simulink model "Aearial_Inspection_UAV_Simulation"  (R2023a)
settings: Solver=daessc  StartTime=0.0  StopTime=tf  MaxStep=0.1  MinStep=1e-30  RelTol=1e-4
values from neighbouring files (symbols this model uses):
  arm_start = 0    [InitScript.m]
  X = T*[x0;y0]    [line2circle.m]
undefined symbols (not defined in the file or in its folder): arm_end, DiscIntNeverNeededParam, F, is_gust_active, Light, MIL, Mode, Motor_data, params, Robotic_Arm_ASM_DataFile, Sensor_err, servo_specs, simple_env, stepper, Tm, wind_speed, xStack1, xStack2, Y, Z
libraries: sm_lib x399, nesl_utility x78, simulink x25, dspsrcs4 x16, simulink_extras x8, sharedtransform x7, aerolibwind2 x2, sharedutil x1
(part 12 of 12)

== matlab function Aearial_Inspection_UAV_Simulation/Path Palnner/Arm Guid/Senario 2/senario_2 ==
  data: t input; desired_pos output; desired_psi output
function [desired_pos,desired_psi] = senario_2(t)

desired_psi = [0 0 0];
desired_pos = [0 0 0];


end

== matlab function Aearial_Inspection_UAV_Simulation/Path Palnner/Arm Guid/Senario 3/senario_3 ==
  data: t input; desired_pos output; desired_psi output
function [desired_pos,desired_psi] = senario_3(t)

desired_psi = [0 0 0];
desired_pos = [0 0 0];


end

== matlab function Aearial_Inspection_UAV_Simulation/Path Palnner/Arm Guid/Senario 4/senario_1 ==
  data: t input; desired_pos output; desired_psi output
function [desired_pos,desired_psi] = senario_4(t)

desired_psi = 0;
desired_pos = [0 0 0];


end

== matlab function Aearial_Inspection_UAV_Simulation/Path Palnner/Arm Guid/Senario 5/senario_5 ==
  data: t input; desired_pos output; desired_psi output; ArmMode input; arm_start parameter; uav_pos input; params parameter
function [desired_pos, desired_psi] = senario_5(t, ArmMode, arm_start, uav_pos, params)
x = uav_pos(1)+0.03;
y = uav_pos(2);
z = uav_pos(3);

start_z = 0.35;
start_x = 1;


lift_up_time = params.t_arm_lift_up;
wait_time    = params.t_arm_wait;
forward_time = params.t_arm_forward_time;
keep_time = params.t_inspection;
backward_time = params.t_probe_backward;
down_time = params.t_probe_down;

if ArmMode == 1
    t = t - arm_start;
    desired_psi = 0;
    if(t<lift_up_time)
        desired_pos = [start_x -y t*(-z-start_z)/lift_up_time+start_z];
    elseif (t < lift_up_time + wait_time)
        desired_pos = [start_x -y -z];
    elseif (t<forward_time+lift_up_time + wait_time)
        t = t - lift_up_time - wait_time;
        desired_pos = [t*(-x-start_x)/forward_time+start_x -y -z];
    elseif t <= forward_time+lift_up_time + wait_time + keep_time
        desired_pos = [-x -y -z+0.007];
    elseif t <= forward_time+lift_up_time + wait_time + keep_time + backward_time
        t = t - (forward_time+lift_up_time + wait_time + keep_time);
        desired_pos = [t*(x+start_x)/backward_time-x -y -z+0.01];
    else
        t = t - (forward_time+lift_up_time + wait_time + keep_time + backward_time);
        t = min(t, down_time);
        desired_pos = [start_x -y t*(z+start_z)/down_time-z];
    end
else
    desired_psi = 0;
    desired_pos = [0. 0 0];
end
end

== matlab function Aearial_Inspection_UAV_Simulation/Controller/Arm Controller/Enabled Subsystem/Arm Senario 2 ==
  data: t input; y output
function y = Arm_Senario_2(t)
t = (t>5)*(t-5);
y = [90*sin(0.25*2*pi*t) * (t<=4)
     90*sin(0.25*2*pi*(t-5)) * (t>=5 && t<=9)
     90*sin(0.25*2*pi*(t-10)) * (t>=10 && t<=14)
     0
     0
     0];

end

== matlab function Aearial_Inspection_UAV_Simulation/Controller/Arm Controller/Arm and Wrist Inv-kinematics/َArm_Controller ==
  data: Mode input; xd input; Servo_Angles output size=[1 3]; yd input; zd input; UAV_Attitude input; ArmMode input
function Servo_Angles = Servo_Controller(Mode, xd, yd, zd, UAV_Attitude, ArmMode)
if Mode == 5 && ArmMode == 1
r_body_to_arm_point_0 = [0.6351 0.001 .133]';
r_arm_point_0_to_a0   = [0 0 -0.004]';
r_arm_a0_to_a1        = [0 0 0.068]';
r_w2_to_prob_disk     = [0.2133 0 -0.04511]';

L1 = 0.433;
L2 = norm([0.433+0.0645, 0.011]);

T_bL = eul2rotm(UAV_Attitude(3:-1:1)' * pi/180)';

desired_vec = T_bL * ([xd; yd; zd] - r_w2_to_prob_disk);
desired_vec = desired_vec - r_body_to_arm_point_0;
desired_vec = desired_vec - r_arm_point_0_to_a0 - r_arm_a0_to_a1;

xd = desired_vec(1);
yd = desired_vec(2);
zd = desired_vec(3);

xd = max(0.1, xd);

a2_bias = atan(0.011/(0.433+0.0645));

% desired point spheric saturation
rd = norm([xd yd]);
hd = -zd;

if abs((-rd^2-hd^2+L1^2+L2^2)/(2*L1*L2))>1
    temp = [rd hd]./norm([rd hd]);
    temp = temp * sqrt(L1^2+L2^2+2*L1*L2)*.99;
    rd = temp(1);
    hd = temp(2);
end

a0 = atan2(yd, xd) + atan2(0.001, rd);

alpha = acos( (-rd^2-hd^2+L1^2+L2^2)/(2*L1*L2) );
a2 = pi/2 - alpha - a2_bias;

alpha = pi - alpha;
temp = [(L1+L2*cos(alpha)) (-L2*sin(alpha)); (L2*sin(alpha)) (L1+L2*cos(alpha))]^-1*[rd; hd];

temp = atan2(temp(2), temp(1));

a1 = -pi/2 - temp;


Servo_Angles = [a0 a1 a2] * 180/pi;
else
    Servo_Angles = [0 60 60];
end
end

== matlab function Aearial_Inspection_UAV_Simulation/Controller/Arm Controller/Arm and Wrist Inv-kinematics/wrist Controller/Subsystem/MATLAB Function ==
  data: R input; a1 output; a2 output; a3 output
function [a1, a2, a3] = fcn(R)

assert(R(1,1) >= 0, "Arm has been Fucked Up!!!!\n theta2 can not be more than 90 deg")

equal_double = @(a, b, tol) (abs(a-b) < tol) && sign(a) == sign(b);
saturation   = @(a, Min, Max) max(min(a, Max), Min);

a2_1 = acos(R(1,1));
a2_2 = -a2_1;

if R(1,1) == 1
    a1 = atan2(R(2,3), R(2,2))/2;
    a3 = a1;
    a2 = 0;    
else
    a1_1 = asin(saturation(R(2,1)/sin(a2_1), -1, 1));
    a1_2 = asin(saturation(R(2,1)/sin(a2_2), -1, 1));
    
    a3_1 = asin(saturation(R(1,2)/sin(a2_1), -1, 1));
    a3_2 = asin(saturation(R(1,2)/sin(a2_2), -1, 1));
    
    if equal_double(R(1,3), -sin(a2_2)*cos(a3_2),0.01) && equal_double(R(3,1), sin(a2_2)*cos(a1_2), 0.01)
        a1 = a3_2;
        a2 = a2_2;
        a3 = a1_2;
    elseif equal_double(R(1,3), -sin(a2_1)*cos(a3_1),0.01) && equal_double(R(3,1), sin(a2_1)*cos(a1_1),0.01)
        a1 = a1_1;
        a2 = a2_1;
        a3 = a3_1;
    else
        assert(false, "no feasilbe solution");
        a1 = a3_2;
        a2 = a2_2;
        a3 = a1_2;
    end
end
assert(true, "unreachable line on wrist controller");
end

== matlab function Aearial_Inspection_UAV_Simulation/Controller/UAV Controller/      1/MATLAB Function ==
  data: Err_of_Atti input; u input; y output
function y = Saturation_Control_Atti(Err_of_Atti, u)


p_dot_max = 50;
q_dot_max = 50;
r_dot_max = 1;


w_max = [sqrt(1.5*p_dot_max*abs(Err_of_Atti(1)));
         sqrt(1.5*q_dot_max*abs(Err_of_Atti(2)));
         sqrt(1.5*r_dot_max*abs(Err_of_Atti(3)))];

y = min(w_max, max(-w_max,u));

== matlab function Aearial_Inspection_UAV_Simulation/Controller/UAV Controller/C-AAC /C-Alt ==
  data: e_Alt input; v_Alt input; u output; w_alt input
function u = Alt_Controller(e_Alt, v_Alt, w_alt)
a_max = 0.8*9.81;
v_max = min(sqrt(a_max*abs(e_Alt)), 3);

vd = min(2*v_max, max(-2*v_max, w_alt*e_Alt)); 
u = min(a_max, max(-a_max,w_alt*(vd-2*v_Alt))); 


end

== matlab function Aearial_Inspection_UAV_Simulation/Controller/UAV Controller/C-AAC /C-Atti ==
  data: e input size=[3 1]; u output; wp input; wq input; wr input
function u = Atti_Controller(e, wp, wq, wr)
e = reshape(e,[3 1]);

p_dot_max = 80;
q_dot_max = 80;
r_dot_max = 3;


k = [wp 0 0
     0 wq 0
     0 0 wr];

w_dot_max = [p_dot_max;q_dot_max;r_dot_max];

u = min(w_dot_max, max(-w_dot_max,k*e)); 


end

== matlab function Aearial_Inspection_UAV_Simulation/Controller/UAV Controller/C-PC/C-Alt ==
  data: e_Pos input; vd input; v_Pos input; u output; wc_x input
function u = Pos_Controller(e_Pos, vd ,v_Pos, wc_x)
a_max = tand(5)*9.81;
v_max = min(sqrt(a_max*abs(e_Pos)), 5);

vd = min(2*v_max, max(-2*v_max, vd + 0.5*wc_x*e_Pos));
u = min(a_max, max(-a_max, 2*wc_x*(vd-2*v_Pos))); 
end

== matlab function Aearial_Inspection_UAV_Simulation/GPS-INS/IMU/Rotation/angle jump correction/MATLAB Function ==
  data: u input; y output; pre_u input; correctio_bias input; correctio_bias output
function [y, correctio_bias] = fcn(u, pre_u, correctio_bias)
correctio_bias = correctio_bias + 2*180*(abs(u-pre_u) > 1.8*180).*sign(pre_u-u);
y = u + correctio_bias;
end

== matlab function Aearial_Inspection_UAV_Simulation/Path Palnner/UAV_Guid/angle jump correction/MATLAB Function ==
  data: u input; y output; pre_u input; correctio_bias input; correctio_bias output
function [y, correctio_bias] = fcn(u, pre_u, correctio_bias)
correctio_bias = correctio_bias + 2*pi*(abs(u-pre_u) > 1.8*pi).*sign(pre_u-u);
y = u + correctio_bias;
end
